simulink model "Linear"  (R2019b)
settings: Solver=ode113  StartTime=0.0  StopTime=50  FixedStep=0.001  RelTol=1e-5
values from neighbouring files (symbols this model uses):
  Gam = 2*diag([1 1])    [Main_Linear.m]
  kp = 3    [Main_Linear.m]
  signkp = sign(kp)    [Main_Linear.m]
  theta = [0;0]    [Main_Linear.m]
libraries: cstblocks x2
settings Model: Creator=Thilo  LastModifiedBy=Thilo

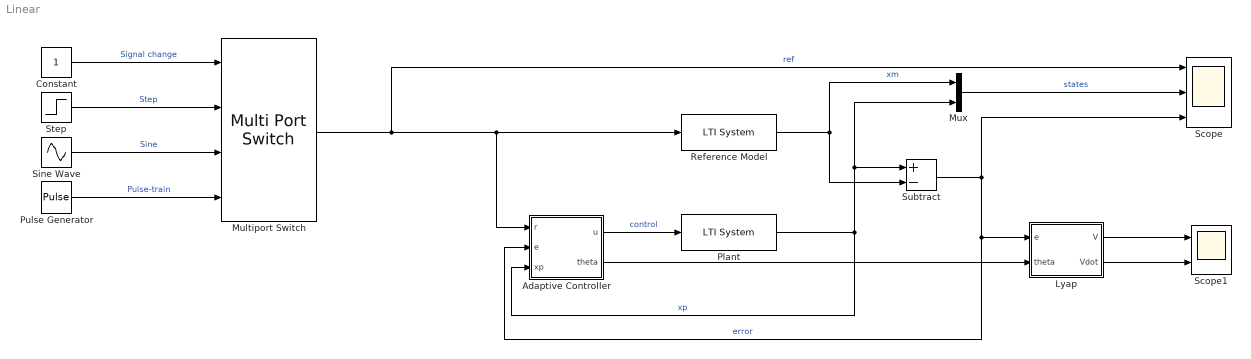
== system Linear ==
  Adaptive Controller : Subsystem
  Constant : Constant
  Lyap : MATLAB Function  TreatAsAtomicUnit=on
  Multiport Switch : MultiPortSwitch
  Mux : Mux  Inputs=2
  Plant : cstblocks/LTI System  sys=G  IC=[0]
  Pulse Generator : DiscretePulseGenerator  PulseType=Time based  Amplitude=4  Period=10  PulseWidth=50
  Reference Model : cstblocks/LTI System  sys=M  IC=[0]
  Scope : Scope  NumInputPorts=3
  Scope1 : Scope  NumInputPorts=2
  Sine Wave : Sin  Amplitude=0.5  SampleTime=0
  Step : Step  Time=0  After=4  SampleTime=0
  Subtract : Sum  Inputs=+-
  wires:
  Multiport Switch/1 -> Scope/1, Reference Model/1, Adaptive Controller/1(r)  "ref"
  Sine Wave/1 -> Multiport Switch/3  "Sine"
  Pulse Generator/1 -> Multiport Switch/4  "Pulse-train"
  Constant/1 -> Multiport Switch/1  "Signal change"
  Step/1 -> Multiport Switch/2  "Step"
  Reference Model/1 -> Mux/1, Subtract/2  "xm"
  Adaptive Controller/1(u) -> Plant/1  "control"
  Plant/1 -> Subtract/1, Mux/2, Adaptive Controller/3(xp)  "xp"
  Mux/1 -> Scope/2  "states"
  Subtract/1 -> Scope/3, Lyap/1(e), Adaptive Controller/2(e)  "error"
  Adaptive Controller/2(theta) -> Lyap/2(theta)
  Lyap/1(V) -> Scope1/1
  Lyap/2(Vdot) -> Scope1/2

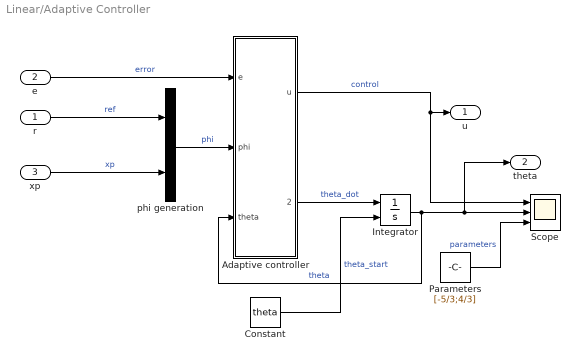
== system Linear/Adaptive Controller ==
  r : Inport
  e : Inport  Port=2
  xp : Inport  Port=3
  Adaptive controller : MATLAB Function  TreatAsAtomicUnit=on
  Constant : Constant  Value=theta
  Integrator : Integrator  InitialConditionSource=external  InitialCondition=[0;0;0]
  Parameters : Constant  Value=[-5/3;4/3]
  Scope : Scope  NumInputPorts=3
  phi generation : Concatenate
  u : Outport
  theta : Outport  Port=2
  wires:
  r/1 -> phi generation/1  "ref"
  xp/1 -> phi generation/2  "xp"
  Integrator/1 -> Adaptive controller/3(theta), theta/1, Scope/2  "theta"
  phi generation/1 -> Adaptive controller/2(phi)  "phi"
  e/1 -> Adaptive controller/1(e)  "error"
  Adaptive controller/1(u) -> Scope/1, u/1  "control"
  Constant/1 -> Integrator/2  "theta_start"
  Adaptive controller/2(thetad) -> Integrator/1  "theta_dot"
  Parameters/1 -> Scope/3  "parameters"

== matlab function Linear/Lyap ==
  data: e input; theta input; V output; kp parameter; Gam parameter; Vdot output
function [V,Vdot] = fcn(e,theta,kp, Gam)
% True parameters
theta_star = [4/3;-5/3];
% Parameter error vector
theta_tilde = theta-theta_star;
% Computation of Lyapunov-like function possible due to knownledge of true
% paramters
V = 0.5*e^2 + 0.5*abs(kp)*theta_tilde'*inv(Gam)*theta_tilde;
% Computation of derivative of Lyapunov-like function
Vdot = -4*e^2;

== matlab function Linear/Adaptive Controller/Adaptive controller ==
  data: e input; phi input; u output; theta input; thetad output; signkp parameter; Gam parameter
function [u,thetad] = fcn(e,phi,theta,signkp,Gam)
% Control
u = theta'*phi;
% Adpative Law
thetad = -signkp*e*Gam*phi;
% thetad = 0;
